simulink model "upcounter"  (R2017b)
settings: Solver=VariableStepAuto  StartTime=0.0  StopTime=10.0  RelTol=1e-3
settings Model: Creator=BCAYR5W  LastModifiedBy=BCAYR5W

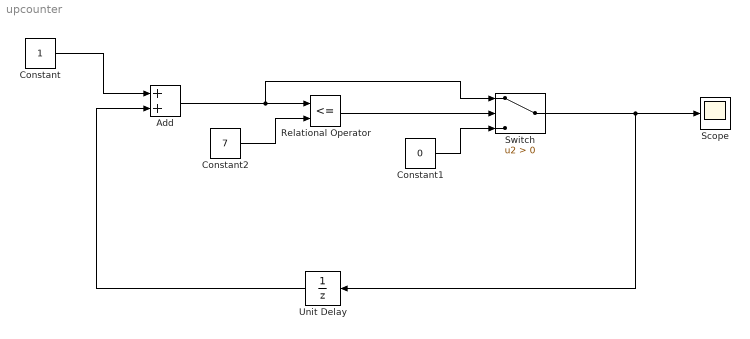
== system upcounter ==
  Add : Sum
  Constant : Constant
  Constant1 : Constant  Value=0
  Constant2 : Constant  Value=7
  Relational Operator : RelationalOperator  Operator=<=  OutDataTypeStr=boolean  RndMeth=Simplest
  Scope : Scope
  Switch : Switch  Criteria=u2 > Threshold
  Unit Delay : UnitDelay  InitialCondition=-1  SampleTime=-1
  wires:
  Constant/1 -> Add/1
  Unit Delay/1 -> Add/2
  Relational Operator/1 -> Switch/2
  Switch/1 -> Scope/1, Unit Delay/1
  Add/1 -> Switch/1, Relational Operator/1
  Constant2/1 -> Relational Operator/2
  Constant1/1 -> Switch/3
